simulink model "case_b"  (R2019b)
settings: Solver=VariableStepAuto  StartTime=0.0  StopTime=time  RelTol=1e-3
values from neighbouring files (symbols this model uses):
  beta = 0.1    [parameters.m]
  Gs = tf(1, [1 3 3 1 0])    [parameters.m]
  half_time = time/2    (= 250)    [parameters.m]
  Kc = 0.56    [parameters.m]
  tauD = 0.3    [parameters.m]
  tauI = 8    [parameters.m]
  time = 500    [parameters.m]
libraries: simulink x2
settings Model: Creator=adityaaaap  LastModifiedBy=adityaaaap

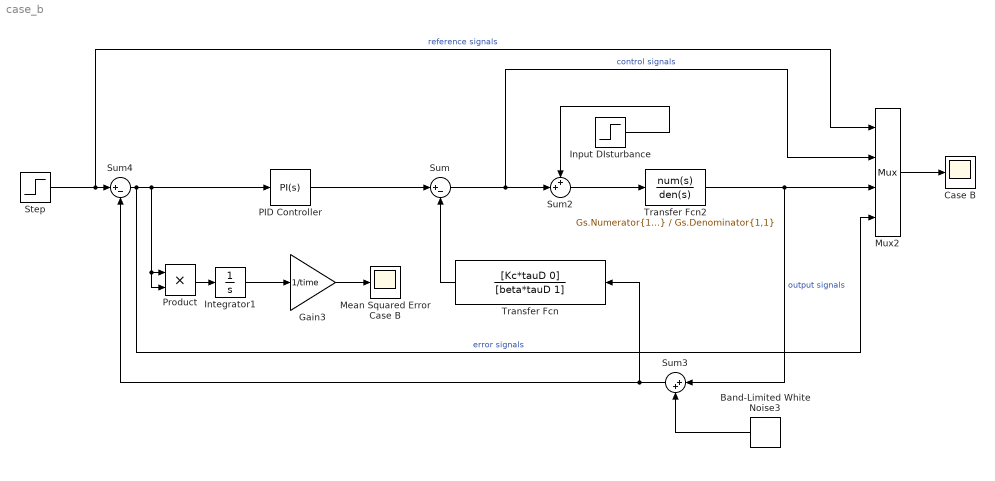
== system case_b ==
  Band-Limited White Noise3 : simulink/Sources/Band-Limited White Noise  Cov=[0.001]  Ts=0.1  seed=[23341]
  Case B : Scope
  Gain3 : Gain  Gain=1/time
  Input DIsturbance : Step  Time=half_time  After=-3  SampleTime=0
  Integrator1 : Integrator
  Mean Squared Error Case B : Scope
  Mux2 : Mux
  PID Controller : simulink/Continuous/PID Controller  Controller=PI  Form=Parallel  TimeDomain=Continuous-time  SampleTime=-1  IntegratorMethod=Forward Euler  FilterMethod=Forward Euler  ControllerParametersSource=internal  P=Kc  I=Kc/tauI  D=Kc*tauD  UseFilter=on  N=1/(0.1*tauD)  TunerSelectOption=Transfer Function Based (PID Tuner App)  InitialConditionSource=internal  InitialConditionForIntegrator=0  InitialConditionForFilter=0  DifferentiatorICPrevScaledInput=0  ExternalReset=none  TrackingMode=off  Kt=1  LimitOutput=off  UpperSaturationLimit=inf  LowerSaturationLimit=-inf  LinearizeAsGain=on  AntiWindupMode=none  Kb=1  POutMin=[]  POutMax=[]  IOutMin=[]  IOutMax=[]  DOutMin=[]  DOutMax=[]  NOutMin=[]  NOutMax=[]  SumOutMin=[]  SumOutMax=[]  SaturationOutMin=[]  SaturationOutMax=[]  PParamMin=[]  PParamMax=[]  IParamMin=[]  IParamMax=[]  DParamMin=[]  DParamMax=[]  NParamMin=[]  NParamMax=[]  KbParamMin=[]  KbParamMax=[]  KtParamMin=[]  KtParamMax=[]  KbOutMin=[]  KbOutMax=[]  KtOutMin=[]  KtOutMax=[]  IntegratorOutMin=[]  IntegratorOutMax=[]  FilterOutMin=[]  FilterOutMax=[]  SumI1OutMin=[]  SumI1OutMax=[]  SumI2OutMin=[]  SumI2OutMax=[]  SumI3OutMin=[]  SumI3OutMax=[]  SumI4OutMin=[]  SumI4OutMax=[]  SumDOutMin=[]  SumDOutMax=[]  DifferentiatorOutMin=[]  DifferentiatorOutMax=[]  FilterDiffOutCoefMin=[]  FilterDiffOutCoefMax=[]  ReciprocalOutMin=[]  ReciprocalOutMax=[]  SumDenOutMin=[]  SumDenOutMax=[]  SumNumOutMin=[]  SumNumOutMax=[]  DivideOutMin=[]  DivideOutMax=[]  IntegratorContinuousStateAttributes=''  IntegratorStateMustResolveToSignalObject=off  IntegratorRTWStateStorageClass=Auto  FilterContinuousStateAttributes=''  FilterStateMustResolveToSignalObject=off  FilterRTWStateStorageClass=Auto  ParallelPVariant=InternalParameters  IdealPVariant=Disabled  IVariant=InternalParameters  DVariant=Disabled  IntegratorVariant=Continuous  SatVariant=Disabled  AWVariant=Passthrough  PCopyVariant=Disabled  TRVariant=Disabled  FdbkBlocksVariant=Forward  IdealPFdbkVariant=Disabled  SatFdbkVariant=Disabled  DerivativeFilterVariant=Disabled  NVariant=Disabled  NCopyVariant=Disabled_SignalSpec  FilterICVariant=Disabled  IntegratorICVariant=InternalICs  ExternalResetVariant=Disabled  TRSumVariant=Passthrough  SumFdbkVariant=Disabled  SumVariant=Sum_PI
  Product : Product
  Step : Step  Time=0  After=6  SampleTime=0.1
  Sum : Sum  Inputs=|+-
  Sum2 : Sum  Inputs=++|
  Sum3 : Sum  Inputs=|++
  Sum4 : Sum  Inputs=|+-
  Transfer Fcn : TransferFcn  Numerator=[Kc*tauD 0]  Denominator=[beta*tauD 1]
  Transfer Fcn2 : TransferFcn  Numerator=Gs.Numerator{1,1}  Denominator=Gs.Denominator{1,1}
  wires:
  Step/1 -> Mux2/1, Sum4/1  "reference signals"
  Mux2/1 -> Case B/1
  Band-Limited White Noise3/1 -> Sum3/2
  Product/1 -> Integrator1/1
  Integrator1/1 -> Gain3/1
  Gain3/1 -> Mean Squared Error Case B/1
  Transfer Fcn2/1 -> Mux2/3, Sum3/1  "output signals"
  Sum3/1 -> Sum4/2, Transfer Fcn/1
  Sum/1 -> Mux2/2, Sum2/2  "control signals"
  Transfer Fcn/1 -> Sum/2
  PID Controller/1 -> Sum/1
  Input DIsturbance/1 -> Sum2/1
  Sum2/1 -> Transfer Fcn2/1
  Sum4/1 -> Mux2/4, PID Controller/1, Product/2, Product/1  "error signals"
